simulink model "exercise02"  (R2022a)
settings: Solver=FixedStepAuto  StartTime=0.0  StopTime=10  FixedStep=0.01  RelTol=1e-3
settings Model: Creator=ac133867  LastModifiedBy=cunis
settings DebuggingCC: UnconnectedInputMsg=warning  UnconnectedOutputMsg=warning  UnconnectedLineMsg=warning
settings RTWCC: DLArmComputeVersion=19.05

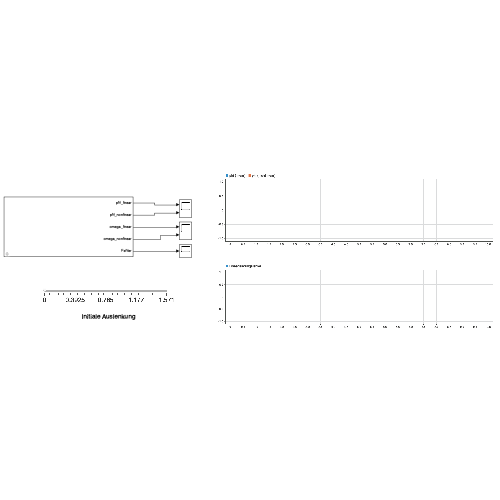
[thumbnail: Simulink's stored preview of the top-level diagram]
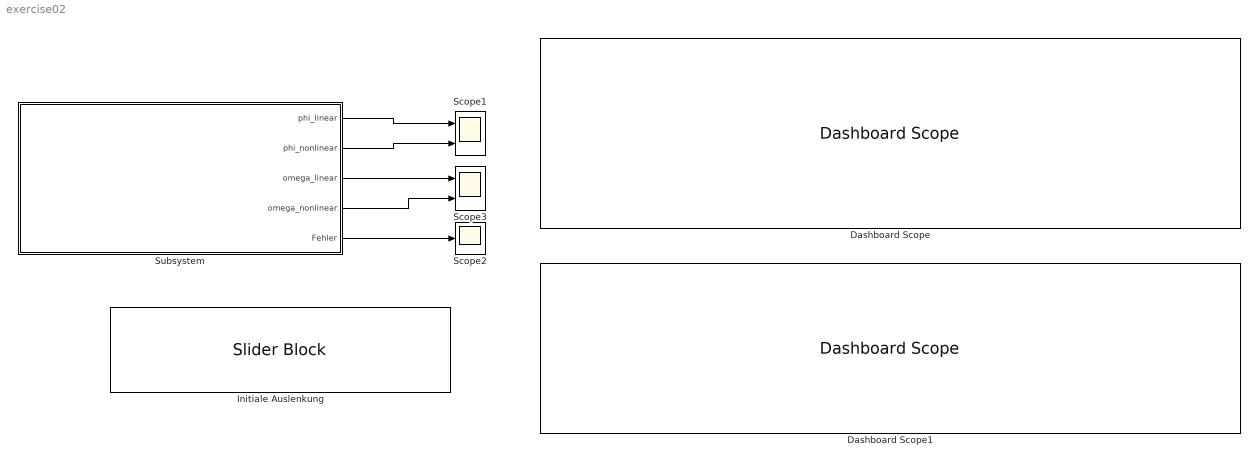
== system exercise02 ==
  Dashboard Scope : DashboardScope
  Dashboard Scope1 : DashboardScope
  Initiale Auslenkung : SliderBlock  LabelPosition=Hide  ScaleMax=1.570796326794897
  Scope1 : Scope  NumInputPorts=2
  Scope2 : Scope
  Scope3 : Scope  NumInputPorts=2
  Subsystem : Subsystem
      mask DialogControl Control2 Prompt: Simulate nonlinear and linear dynamics of a pendulum. Equilibrium point is (0,0)^T
  wires:
  Subsystem/1(phi_linear) -> Scope1/1
  Subsystem/2(phi_nonlinear) -> Scope1/2
  Subsystem/3(omega_linear) -> Scope3/1
  Subsystem/4(omega_nonlinear) -> Scope3/2
  Subsystem/5(Fehler) -> Scope2/1

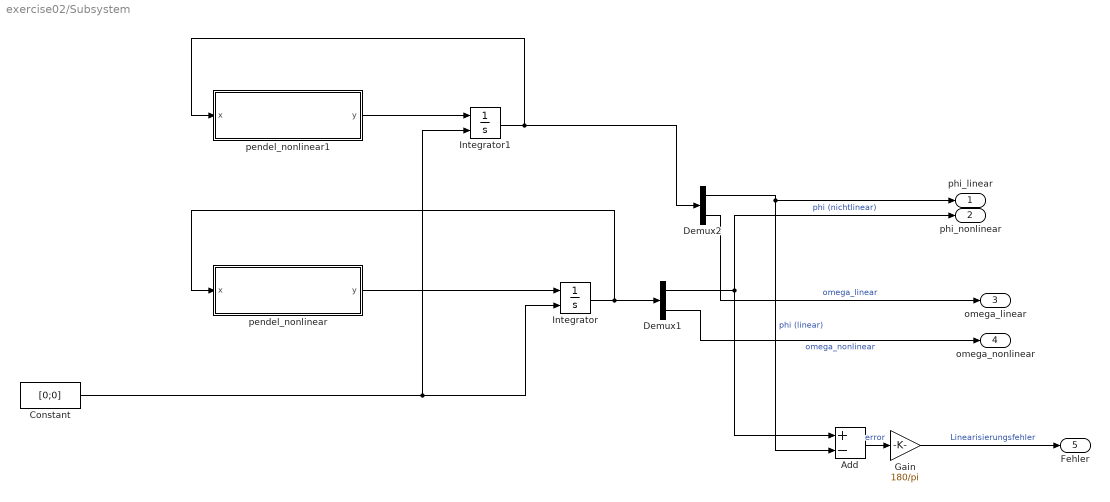
== system exercise02/Subsystem ==
  Add : Sum  Inputs=+-
  Constant : Constant  Value=[0;0]
  Demux1 : Demux  Outputs=2
  Demux2 : Demux  Outputs=2
  Gain : Gain  Gain=180/pi
  Integrator : Integrator  InitialConditionSource=external  InitialCondition=[45*pi/180;0]
  Integrator1 : Integrator  InitialConditionSource=external  InitialCondition=[45*pi/180;0]
  pendel_nonlinear : MATLAB Function  TreatAsAtomicUnit=on
  pendel_nonlinear1 : MATLAB Function  TreatAsAtomicUnit=on
  phi_linear : Outport
  phi_nonlinear : Outport  Port=2
  omega_linear : Outport  Port=3
  omega_nonlinear : Outport  Port=4
  Fehler : Outport  Port=5
  wires:
  Demux1/1 -> phi_nonlinear/1, Add/1  "phi (nichtlinear)"
  Demux2/1 -> phi_linear/1, Add/2  "phi (linear)"
  Integrator/1 -> Demux1/1, pendel_nonlinear/1(x)
  Constant/1 -> Integrator1/2, Integrator/2
  pendel_nonlinear/1(y) -> Integrator/1
  pendel_nonlinear1/1(y) -> Integrator1/1
  Demux1/2 -> omega_nonlinear/1  "omega_nonlinear"
  Integrator1/1 -> Demux2/1, pendel_nonlinear1/1(x)
  Add/1 -> Gain/1  "error"
  Demux2/2 -> omega_linear/1  "omega_linear"
  Gain/1 -> Fehler/1  "Linearisierungsfehler"

== matlab function exercise02/Subsystem/pendel_nonlinear ==
  data: x input; y output
function y = pendel_nonlinear(x)


c = 0.2;
l = 1;
m = 1;
g = 9.81;

y = [0 1; 0 -c/m]*x+ [0; -g/l*sin(x(1))];

== matlab function exercise02/Subsystem/pendel_nonlinear1 ==
  data: x input; y output
function y = pendel_linear(x)


c = 0.2;
l = 1;
m = 1;
g = 9.81;

y =  [              0,    1;
     -g/l, -c/m]*x;
